simulink model "control"  (R2020a)
settings: Solver=FixedStepDiscrete  StartTime=0.0  StopTime=1  FixedStep=0.0005  RelTol=1e-3  EnableMultiTasking=on
undefined symbols (not defined in the file): acc_calmax1, acc_calmax2, acc_calmin1, acc_calmin2, akemancanshu, bre, bre_calmax, bre_calmin, ecucoder_acal, I_AN01_5K1, I_AN03_5V, I_AN04_5V, kd, ki, kp, leftmax, O_SW06_HS1A, rightmax, T_add, T_del, tiaoshi, zhiling
libraries: ec5744lib x252, canmsglib x92, simulink x5
(part 8 of 9)

== matlab function control/Subsystem/run/ctrl/Subsystem1/control_strategy/限滑/MPC/MPC/MPC左后/MPC_function ==
  data: x_k input; u_k output; U_init input
function u_k= Prediction(x_k,U_init)
% 定义状态矩阵 A, n*n 矩阵
A = 0;
% 定义输入矩阵 B, n*p 矩阵
R=0.2032;
FN=2058;
K=6.89;
B = R/(FN*K);
p = size(B,2);
% 定义Q矩阵，n*n 矩阵
Q = 100;
% 定义F矩阵，n*n 矩阵
F = 100;
% 定义R矩阵，p*p 矩阵
R = 1;
% 定义迭代次数和学习率
maxIterations = 5;
learningRate = 0.3;
N=5;%预测区间
n=size(A,1); % A是n*n矩阵,得到n
p=size(B,2); % B是n*p矩阵,得到p
M=[eye(n);zeros(N*n,n)]; % 初始化M矩阵,M矩阵是(N+1)n*n的
D=[0.17;zeros(N*n,n)];
C=zeros((N+1)*n,N*p); % 初始化C矩阵,这一步令它有(N+1)n*NP个0

% 定义M和C
tmp=eye(n); % 定义一个n*n 的 I 矩阵
    for i=1:N % 循环,i从1到N
        rows =i*n+(1:n); %定义当前行数,从i*n开始，共n行
        C(rows,:)=[tmp*B,C(rows-n, 1:end-p)]; %将c矩阵填满
        tmp= A*tmp; %每一次将tmp左乘一次A
        M(rows,:)=tmp; %将M矩阵写满
         D(rows,:)=0.17;
    end
    % 定义Q_bar和R_bar
    Q_bar = kron(eye(N),Q);
    Q_bar = blkdiag(Q_bar,F);
    R_bar = kron(eye(N),R);
    % 计算G,E,H
    G=M'*Q_bar*M; % G: n*n
    E=C'*Q_bar*M; % E: NP*n
    H=C'*Q_bar*C+R_bar; % NP*NP
 J=(D'*Q_bar*C)';
 L=E*x_k+J;
 U = U_init*ones(N*p,1); % NP x 1
%  options = optimoptions('quadprog', 'Algorithm', 'active-set');
%  U_k = quadprog(H,L, [], [], [], [], 0*ones(5,1), 1100*ones(5,1), 100*ones(5,1), options);
    % 梯度下降法求解最优二次规划问题
    G=size(U,1);
    S=zeros(G*maxIterations,1);
    for i = 1:maxIterations
        % 计算目标函数的梯度
        gradient = 2*H*U + 2*L;
        % 更新变量 U，并保持在 [0, 1100] 范围内
        U = U - learningRate * gradient;
        U = max(U, 0);
        U = min(U, 1100);
        O=(i-1)*maxIterations+(1:maxIterations);
        S(O,1)=U;
    end

 u_k = S(1:p,1); % 取第一个结果
end

== matlab function control/Subsystem/run/ctrl/Subsystem1/control_strategy/限滑/PID限滑/pid限滑与ABS ==
  data: slip input; throttle output; slip_ratio_limit input; brake output; u input
function [throttle, brake] = carPIDWithSlipControl(slip, slip_ratio_limit,u)
    % 赛车PID控制器参数
    kp = 0.2;
    ki = 0.1;
    kd = 0.01;
    
    % 状态变量
    persistent integral previous_error i
    
    % 初始化状态变量
    if isempty(integral)
        integral = 0;
        previous_error = 0;
        i=0;
    end
    
    % PID控制器计算
    error = 0.2 - slip;
    integral = integral + error*0.02;
    derivative = (error - previous_error)/0.02;
    
   k = kp * error + ki * integral + kd * derivative;
    if i<100
    
        output = u+k*u;
        if output>2000
            output=2000;
        end
    else
        output=u;
    end
    % 根据滑移率限制输出
  
    if slip > slip_ratio_limit
        brake = 0;%output;
        throttle = 0;
    else
        brake = 0;
        throttle = output;
    end
    
    % 保存上一个误差用于下次计算
    previous_error = error;

    i=i+1;
end

== matlab function control/Subsystem/run/ctrl/Subsystem1/control_strategy/限滑/PID限滑/pid限滑与ABS1 ==
  data: slip input; throttle output; slip_ratio_limit input; brake output; u input
function [throttle, brake] = carPIDWithSlipControl(slip, slip_ratio_limit,u)
    % 赛车PID控制器参数
    kp = 0.2;
    ki = 0.1;
    kd = 0.01;
    
    % 状态变量
    persistent integral previous_error i
    
    % 初始化状态变量
    if isempty(integral)
        integral = 0;
        previous_error = 0;
        i=0;
    end
    
    % PID控制器计算
    error = 0.2 - slip;
    integral = integral + error*0.02;
    derivative = (error - previous_error)/0.02;
    
   k = kp * error + ki * integral + kd * derivative;
    if i<100
    
        output = u+k*u;
        if output>2000
            output=2000;
        end
    else
        output=u;
    end
    % 根据滑移率限制输出
  
    if slip > slip_ratio_limit
        brake = 0;%output;
        throttle = 0;
    else
        brake = 0;
        throttle = output;
    end
    
    % 保存上一个误差用于下次计算
    previous_error = error;
    i=i+1;
end

== matlab function control/Subsystem/run/ctrl/Subsystem1/control_strategy/限滑/PID限滑/pid限滑与ABS2 ==
  data: slip input; throttle output; slip_ratio_limit input; brake output; u input
function [throttle, brake] = carPIDWithSlipControl(slip, slip_ratio_limit,u)
    % 赛车PID控制器参数
    kp = 0.2;
    ki = 0.1;
    kd = 0.01;
    
    % 状态变量
    persistent integral previous_error i
    
    % 初始化状态变量
    if isempty(integral)
        integral = 0;
        previous_error = 0;
        i=0;
    end
    
    % PID控制器计算
    error = 0.2 - slip;
    integral = integral + error*0.02;
    derivative = (error - previous_error)/0.02;
   k = kp * error + ki * integral + kd * derivative;
    if i<100
    
        output = u+k*u;
        if output>2000
            output=2000;
        end
    else
        output=u;
    end
    % 根据滑移率限制输出
  
    if slip > slip_ratio_limit
        brake = 0;%output;
        throttle = 0;
    else
        brake = 0;
        throttle = output;
    end
    
    % 保存上一个误差用于下次计算
    previous_error = error;
    i=i+1;
end

== matlab function control/Subsystem/run/ctrl/Subsystem1/control_strategy/限滑/PID限滑/pid限滑与ABS3 ==
  data: slip input; throttle output; slip_ratio_limit input; brake output; u input
function [throttle, brake] = carPIDWithSlipControl(slip, slip_ratio_limit,u)
    % 赛车PID控制器参数
    kp = 0.2;
    ki = 0.1;
    kd = 0.01;
    
    % 状态变量
    persistent integral previous_error i
    
    % 初始化状态变量
    if isempty(integral)
        integral = 0;
        previous_error = 0;
        i=0;
    end
    
    % PID控制器计算
    error = 0.2 - slip;
    integral = integral + error*0.02;
    derivative = (error - previous_error)/0.02;
    
   k = kp * error + ki * integral + kd * derivative;
    if i<100
    
        output = u+k*u;
        if output>2000
            output=2000;
        end
    else
        output=u;
    end
    % 根据滑移率限制输出
  
    if slip > slip_ratio_limit
        brake =0;% output;
        throttle = 0;
    else
        brake = 0;
        throttle = output;
    end
    
    % 保存上一个误差用于下次计算
    previous_error = error;
    i=i+1;
end

== matlab function control/Subsystem/Tx/TX控制器/速度/189左后/MATLAB Function5 ==
  data: v input; y output; angle input; vz input; model input
function y = fcn(v, angle, vz,model)
if(angle>3||angle<-3)&&model==3%4650000,4870000,4741002
    y=vz*594.06;
else
    y = v;
end

== matlab function control/Subsystem/run/ctrl/Subsystem1/control_strategy/限滑/PID限滑/计算油压 ==
  data: y1 input; p1 output; y2 input; y3 input; y4 input; p2 output; p3 output; p4 output
function [p1,p2,p3,p4]= fcn(y1,y2,y3,y4)
S=0.000491;
%p1 p2 p3 p4分别是左前、右前、左后、右后油压
p1=y1/(0.8*S)/1000;
p2=y2/(0.8*S)/1000;
p3=y3/(0.4*S)/1000;
p4=y4/(0.4*S)/1000;
% if p1<0
%     p1=0;
%     end
% if p2<0
%     p2=0;
%     end
% if p3<0
%     p3=0;
%     end
% if p4<0
%     p4=0;
% end

== matlab function control/Subsystem/run/ctrl/Subsystem1/control_strategy/限滑/Subsystem1/MATLAB Function2 ==
  data: u input; y output; mpc input; pid input; slip input; model input
function y = fcn(u,mpc,pid,slip,model)
if slip>0.8&&model~=6
    y=pid;
elseif slip>0.165&&slip<0.17
        y=mpc;
else
        y=u;
end
end

== matlab function control/Subsystem/run/ctrl/Subsystem1/control_strategy/限滑/Subsystem1/MATLAB Function3 ==
  data: u input; y output; mpc input; pid input; slip input; model input
function y = fcn(u,mpc,pid,slip,model)
if slip>0.8&&model~=6
    y=pid;
elseif slip>0.169&&slip<0.17
        y=mpc;
else
        y=u;
end
end

== matlab function control/Subsystem/run/ctrl/Subsystem1/control_strategy/限滑/Subsystem1/MATLAB Function4 ==
  data: u input; y output; mpc input; pid input; slip input; model input
function y = fcn(u,mpc,pid,slip,model)
if slip>0.8&&model~=6
    y=pid;
elseif slip>0.165&&slip<0.17
        y=mpc;
else
        y=u;
end
end

== matlab function control/Subsystem/run/ctrl/Subsystem1/control_strategy/限滑/Subsystem1/MATLAB Function5 ==
  data: u input; y output; mpc input; pid input; slip input; model input
function y = fcn(u,mpc,pid,slip,model)
if slip>0.8&&model~=6
    y=pid;
elseif slip>0.165&&slip<0.17
        y=mpc;
else
        y=u;
end
end

== matlab function control/Subsystem/Tx/TX控制器/速度1/184左前/MATLAB Function7 ==
  data: T input; y output; wurenyouya input; youya input; enable input; enable_1 input
function y = fcn(T, wurenyouya,youya, enable, enable_1)
 y = 0;
if wurenyouya>10||youya>500
    y = T;
else
    y=0;
end
if enable==0
    y=0;
end

== matlab function control/Subsystem/run/滑移率计算 ==
  data: vyouhou input; slipyuohou output; vyouqian input; vzouhou input; vzuoqian input; v input; slipyouqian output; slipzuohou output; slipzuoqian output; vmin input
function [slipyuohou,slipyouqian,slipzuohou,slipzuoqian] = fcn(vyouhou,vyouqian,vzouhou,vzuoqian,v,vmin)

    v1=vmin;
if v<0.1
    v1 = vmin;
else
    v1 = v;
end
slipyuohou= (vyouhou - v1) / vyouhou;
slipzuohou= (vzouhou - v1) / vzouhou;
slipyouqian= (vyouqian - v1) / vyouqian;
slipzuoqian= (vzuoqian - v1) / vzuoqian;
end

== matlab function control/Subsystem/Tx/TX控制器/速度1/188右后/MATLAB Function7 ==
  data: v input; youren input; T output; model input
function T = fcn(v,youren, model)
% if a>5
%     y = u;
% elseif a>3&&a<5
%     y=1200;
% else
%     y=800;
% end

if model==0||model==9||model==10   %有人模式，调试模式
    T=youren;
else                    %无人模式
   if v<6000*1.88e-3
     T=2100;
    elseif v>11000*1.88e-3
        T=800;
    else
        T=1100;
   end
end

== matlab function control/Subsystem/run/kalman_filter2 ==
  data: a_k_1 input; y output; v_k_1 input; v_k input; V_MIN input; model input
function y = fcn(a_k_1,v_k_1,v_k,V_MIN, model)
A=1;
H=1;
% x_real=v_k_1+0.02*a_k_1;%首先给出一个相应的估计值
% z=0;
% w=0;
% v=0;
% %%噪声信号
%     w=1*randn;
%     v=1*randn;
% %%状态方程
%     x_real=A*v_k_1+0.02*a_k_1+w;
% %%观测方程
%     z=H*x_real+v;
% persistent xhat;
%      % 初始化状态变量
%     if isempty(xhat)
%         xhat = V_MIN;
%     end

    z=H*v_k;
%%kalman_filter  根据上述得观测值来不断更新  
xhat=v_k;
xhat=v_k_1+0.02*a_k_1;%先验估计
Q=1;
R=0.01;
Pk=1;
Pk_bar=0;%先验协方差

    xhat_=v_k_1+0.02*a_k_1;%先验估计
    Pk_bar=A*Pk*A'+Q;
    Kk=Pk_bar*H'/(H*Pk_bar*H'+R);
    xhat= xhat_+ Kk*(z-H* xhat_);%最优估计值
    Pk=(1-Kk*H)*Pk_bar;
if v_k<0.1||model==0||model==9
    y=V_MIN;%即转轮时不使用惯导信息
elseif abs(xhat-v_k)>0.5
    y=v_k;
else
    y = xhat;
end
end

== matlab function control/Subsystem/Tx/TX控制器/速度/189左后/MATLAB Function6 ==
  data: v input; T output; a input
function T = fcn(v,a)
% if a>5
%     y = u;
% elseif a>3&&a<5
%     y=1200;
% else
%     y=800;
% end

if v<6000*1.88e-3
    T=2100;
elseif v>11000*1.88e-3
    T=800;
else
    T=1100;
end

== matlab function control/Subsystem/Tx/TX控制器/速度1/188右后/MATLAB Function6 ==
  data: T input; y output; wurenyouya input; youya input; enable input; enable_1 input
function y = fcn(T, wurenyouya,youya, enable, enable_1)
 y = 0;
if wurenyouya>10||youya>500
    y = T;
else
    y=0;
end
if enable==0
    y=0;
end

== matlab function control/Subsystem/Tx/TX控制器/速度1/189左后/MATLAB Function7 ==
  data: T input; y output; wurenyouya input; youya input; enable input; enable_1 input
function y = fcn(T, wurenyouya,youya, enable, enable_1)
 y = 0;
if wurenyouya>10||youya>500
    y = T;
else
    y=0;
end
if enable==0
    y=0;
end

== matlab function control/Subsystem/Tx/TX控制器/速度1/185右前/MATLAB Function7 ==
  data: T input; y output; wurenyouya input; youya input; enable input; enable_1 input
function y = fcn(T, wurenyouya,youya, enable, enable_1)
 y = 0;
if wurenyouya>10||youya>500
    y = T;
else
    y=0;
end
if enable==0
    y=0;
end

== matlab function control/Subsystem/Tx/TX控制器/速度1/184左前/能量回收功率限制/MATLAB Function ==
  data: youya input; T output; model input; status input; wurenyouya input
function T = fcn(youya, model, status, wurenyouya)
    if model == 0||model==10  %有人模式
        if youya>500
            T = -(youya-500)/4;%最大反扭1000
            if youya>4500
                T = -1000;
            end
        else
            T = 0;
        end
        
    elseif model~=0&&model~=9&&model~=2  %无人模式
        if wurenyouya>10
            T = -wurenyouya
            if status==5
                T=-1000;
            end  
           % T = -(wurenyouya-500)/4;%最大反扭1000
            %if wurenyouya>500&&status==5
             %   T = -1000;
            %end
        else
            T = 0;
        end
    else
        T = 0;
end

== matlab function control/Subsystem/Tx/TX控制器/速度1/184左前/能量回收功率限制/MATLAB Function1 ==
  data: er_T input; T output; Iq input; L_Iq input; L_er_T input
function T = fcn(er_T, Iq, L_Iq,L_er_T)
    if abs(Iq)>abs(L_Iq)
        T = -abs(L_er_T);

    else
        T = -abs(er_T);
    end

== matlab function control/Subsystem/Tx/TX控制器/速度1/188右后/能量回收功率限制/MATLAB Function ==
  data: youya input; T output; model input; status input; wurenyouya input
function T = fcn(youya, model, status, wurenyouya)
    if model == 0||model==10  %有人模式
        if youya>500
            T = -(youya-500)/4;%最大反扭1000
            if youya>4500
                T = -1000;
            end
        else
            T = 0;
        end
        
    elseif model~=0&&model~=9&&model~=2  %无人模式
        if wurenyouya>10
            T = -wurenyouya
        if status==5
                T=-1000;
            end  
           % T = -(wurenyouya-500)/4;%最大反扭1000
            %if wurenyouya>500&&status==5
             %   T = -1000;
            %end
        else
            T = 0;
        end
    else
        T = 0;
end

== matlab function control/Subsystem/Tx/TX控制器/速度1/188右后/能量回收功率限制/MATLAB Function1 ==
  data: er_T input; T output; Iq input; L_Iq input; L_er_T input
function T = fcn(er_T, Iq, L_Iq,L_er_T)
    if abs(Iq)>abs(L_Iq)
        T = -abs(L_er_T);

    else
        T = -abs(er_T);
    end

== matlab function control/Subsystem/Tx/TX控制器/速度/185右前/MATLAB Function2 ==
  data: enable input; enable_1 input; T input; TargetVelocity output; AMK_TorqueLimitPositive output; enable output; errorreset output; blnverteron output; CAN_dbcon output; v input
function [TargetVelocity,AMK_TorqueLimitPositive,enable,errorreset,blnverteron,CAN_dbcon]= fcn(enable,enable_1,T,v)
if (enable_1==0)
    TargetVelocity=0;
    enable=0;
    errorreset=1;
    blnverteron=0;
    CAN_dbcon=0;
    AMK_TorqueLimitPositive=0;
elseif (enable==0 && enable_1==1)
    TargetVelocity=2000;
    enable=1;
    errorreset=0;
    blnverteron=1;
    CAN_dbcon=1;
    AMK_TorqueLimitPositive=0;
elseif (enable==1 && enable_1==1)
    TargetVelocity=2000;
    enable=1;
    errorreset=0;
    blnverteron=1;
    CAN_dbcon=1;
    AMK_TorqueLimitPositive=T;
else
    TargetVelocity=0;
    enable=0;
    errorreset=1;
    blnverteron=0;
    CAN_dbcon=0;
    AMK_TorqueLimitPositive=0;
end

end

== matlab function control/Subsystem/Tx/TX控制器/速度1/189左后/能量回收功率限制/MATLAB Function ==
  data: youya input; T output; model input; status input; wurenyouya input
function T = fcn(youya, model, status, wurenyouya)
    if model == 0||model==10  %有人模式
        if youya>500
            T = -(youya-500)/4;%最大反扭1000
            if youya>4500
                T = -1000;
            end
        else
            T = 0;
        end
        
    elseif model~=0&&model~=9&&model~=2  %无人模式
        if wurenyouya>10
            T = -wurenyouya
            if status==5
                T=-1000;
            end
            
           % T = -(wurenyouya-500)/4;%最大反扭1000
            %if wurenyouya>500&&status==5
             %   T = -1000;
            %end
        else
            T = 0;
        end
    else
        T = 0;
end

== matlab function control/Subsystem/Tx/TX控制器/速度1/189左后/能量回收功率限制/MATLAB Function1 ==
  data: er_T input; T output; Iq input; L_Iq input; L_er_T input
function T = fcn(er_T, Iq, L_Iq,L_er_T)
    if abs(Iq)>abs(L_Iq)
        T = -abs(L_er_T);

    else
        T = -abs(er_T);
    end

== matlab function control/Subsystem/Tx/TX控制器/速度1/185右前/能量回收功率限制/MATLAB Function ==
  data: youya input; T output; model input; status input; wurenyouya input
function T = fcn(youya, model, status, wurenyouya)
    if model == 0||model==10  %有人模式
        if youya>500
            T = -(youya-500)/4;%最大反扭1000
            if youya>4500
                T = -1000;
            end
        else
            T = 0;
        end
        
    elseif model~=0&&model~=9&&model~=2  %无人模式
        if wurenyouya>10
            T = -wurenyouya
        if status==5
                T=-1000;
            end  
           % T = -(wurenyouya-500)/4;%最大反扭1000
            %if wurenyouya>500&&status==5
             %   T = -1000;
            %end
        else
            T = 0;
        end
    else
        T = 0;
end

== matlab function control/Subsystem/Tx/TX控制器/速度1/185右前/能量回收功率限制/MATLAB Function1 ==
  data: er_T input; T output; Iq input; L_Iq input; L_er_T input
function T = fcn(er_T, Iq, L_Iq,L_er_T)
    if abs(Iq)>abs(L_Iq)
        T = -abs(L_er_T);

    else
        T = -abs(er_T);
    end

== matlab function control/Subsystem/run/analog_input/无人意图转译/无人/Subsystem1/Subsystem/MATLAB Function ==
  data: u input; y output; v input; vd input
function y = fcn(u,v,vd)
persistent vv
if isempty(vv)
    vv=0;
end
if v-vd>0.1*v
    y=vv
else
    y=u;
end
vv=u;

== matlab function control/Subsystem/run/analog_input/MATLAB Function6 ==
  data: model input; y output
function y = fcn(model)
if model~=0||model~=10
    y = 1;
else
    y=0;
end

== matlab function control/Subsystem/Tx/TX控制器/速度/185右前/MATLAB Function4 ==
  data: u input; y output; zhidongesc input; zhidongebs input; huanting input
function y = fcn(u,zhidongesc,zhidongebs,huanting)
 y = u*594.06;
if zhidongesc>1800&&zhidongebs==2
    y = u*594.06;
end
if zhidongesc<1500&&zhidongebs==2
    y=0;
end
if huanting~=0
    y=0;
end

== matlab function control/Subsystem/Tx/TX控制器/速度/185右前/MATLAB Function5 ==
  data: v input; y output; angle input; vz input; model input
function y = fcn(v, angle, vz,model)
if(angle>3||angle<-3)&&model==3%4650000,4870000,4741002
    y=vz*594.06;
else
    y = v;
end

== matlab function control/Subsystem/Tx/TX控制器/速度/185右前/MATLAB Function6 ==
  data: v input; T output; a input
function T = fcn(v,a)
% if a>5
%     y = u;
% elseif a>3&&a<5
%     y=1200;
% else
%     y=800;
% end

if v<6000*1.88e-3
    T=2100;
elseif v>11000*1.88e-3
    T=800;
else
    T=1100;
end

== matlab function control/Subsystem/Tx/TX控制器/速度1/184左前/MATLAB Function ==
  data: u input; y output; zhidongesc input; zhidongebs input; huanting input
function y = fcn(u,zhidongesc,zhidongebs,huanting)
 y = u*594.06;
if zhidongesc>1800&&zhidongebs==2
    y = u*594.06;
end
if zhidongesc<1500&&zhidongebs==2
    y=0;
end
if huanting==0
    y=0;
end

== matlab function control/Subsystem/Tx/TX控制器/速度1/184左前/MATLAB Function1 ==
  data: v input; T output; a input
function T = fcn(v,a)
% if a>5
%     y = u;
% elseif a>3&&a<5
%     y=1200;
% else
%     y=800;
% end

if v<6000*1.88e-3
    T=2100;
elseif v>11000*1.88e-3
    T=800;
else
    T=1100;
end

== matlab function control/Subsystem/Tx/TX控制器/速度1/184左前/复位 ==
  data: enable input; enable_1 input; T input; TargetVelocity output; AMK_TorqueLimitPositive output; enable output; errorreset output; blnverteron output; CAN_dbcon output; v input
function [TargetVelocity,AMK_TorqueLimitPositive,enable,errorreset,blnverteron,CAN_dbcon]= fcn(enable,enable_1,T,v)
if (enable_1==0)
    TargetVelocity=0;
    enable=0;
    errorreset=1;
    blnverteron=0;
    CAN_dbcon=0;
    AMK_TorqueLimitPositive=0;
elseif (enable==0 && enable_1==1)
    TargetVelocity=0;
    enable=1;
    errorreset=0;
    blnverteron=1;
    CAN_dbcon=1;
    AMK_TorqueLimitPositive=0;
elseif (enable==1 && enable_1==1)
    TargetVelocity=v;
    enable=1;
    errorreset=0;
    blnverteron=1;
    CAN_dbcon=1;
    AMK_TorqueLimitPositive=T;
else
    TargetVelocity=0;
    enable=0;
    errorreset=1;
    blnverteron=0;
    CAN_dbcon=0;
    AMK_TorqueLimitPositive=0;
end

end

== matlab function control/Subsystem/Tx/TX控制器/速度/184左前/MATLAB Function2 ==
  data: enable input; enable_1 input; T input; TargetVelocity output; AMK_TorqueLimitPositive output; enable output; errorreset output; blnverteron output; CAN_dbcon output; v input
function [TargetVelocity,AMK_TorqueLimitPositive,enable,errorreset,blnverteron,CAN_dbcon]= fcn(enable,enable_1,T,v)
if (enable_1==0)
    TargetVelocity=0;
    enable=0;
    errorreset=1;
    blnverteron=0;
    CAN_dbcon=0;
    AMK_TorqueLimitPositive=0;
elseif (enable==0 && enable_1==1)
    TargetVelocity=2000;
    enable=1;
    errorreset=0;
    blnverteron=1;
    CAN_dbcon=1;
    AMK_TorqueLimitPositive=0;
elseif (enable==1 && enable_1==1)
    TargetVelocity=2000;
    enable=1;
    errorreset=0;
    blnverteron=1;
    CAN_dbcon=1;
    AMK_TorqueLimitPositive=T;
else
    TargetVelocity=0;
    enable=0;
    errorreset=1;
    blnverteron=0;
    CAN_dbcon=0;
    AMK_TorqueLimitPositive=0;
end

end

== matlab function control/Subsystem/Tx/TX控制器/速度1/184左前/MATLAB Function3 ==
  data: v input; y output; angle input; vz input; model input
function y = fcn(v, angle, vz,model)
if(angle>3||angle<-3)&&model==3%4650000,4870000,4741002
    y=vz*594.06;
else
    y = v;
end

== matlab function control/Subsystem/Tx/TX控制器/速度1/184左前/无人模式速度判断 ==
  data: u input; y output; zhidongesc input; zhidongebs input; huanting input
function y = fcn(u,zhidongesc,zhidongebs,huanting)
 y = u*594.06;
if zhidongesc>1800&&zhidongebs==2
    y = u*594.06;
end
if zhidongesc<1500&&zhidongebs==2
    y=0;
end
if huanting~=0
    y=0;
end

== matlab function control/Subsystem/Tx/TX控制器/速度1/184左前/有人无人速度转换 ==
  data: v input; y output; angle input; vz input; model input; zhidong input; T input; vk input
function y = fcn(v, angle, vz,model, zhidong, T, vk)
if model==0||model==9||model==10  %有人模式/无人检查（电气）
    if zhidong==0
       y=20000;
    else 
        y=0;
    end
else                    %无人模式
    if (angle>3||angle<-3)&&model==3 %4650000,4870000,4741002 大角度且八字
        y=vz*594.06;
    elseif T >10
        y=0;
        if vk<1
            y=vz*594.06;
        end
    else
        y = v;  
    end    
end

== matlab function control/Subsystem/Tx/TX控制器/速度1/184左前/有人无人扭矩转换 ==
  data: v input; youren input; T output; model input
function T = fcn(v,youren, model)
% if a>5
%     y = u;
% elseif a>3&&a<5
%     y=1200;
% else
%     y=800;
% end

if model==0||model==9||model==10   %有人模式，调试模式
    T=youren;
else                    %无人模式
   if v<6000*1.88e-3
     T=2100;
    elseif v>11000*1.88e-3
        T=800;
    else
        T=1100;
   end
end

== matlab function control/Subsystem/Tx/TX控制器/速度1/185右前/MATLAB Function ==
  data: u input; y output; zhidongesc input; zhidongebs input
function y = fcn(u,zhidongesc,zhidongebs)
 y = u*594.06;
if zhidongesc>1800&&zhidongebs==2
    y = u*594.06;
end
if zhidongesc<1500&&zhidongebs==2
    y=0;
end

== matlab function control/Subsystem/Tx/TX控制器/速度1/185右前/MATLAB Function1 ==
  data: v input; T output; a input
function T = fcn(v,a)
% if a>5
%     y = u;
% elseif a>3&&a<5
%     y=1200;
% else
%     y=800;
% end

if v<6000*1.88e-3
    T=2100;
elseif v>11000*1.88e-3
    T=800;
else
    T=1100;
end

== matlab function control/Subsystem/Tx/TX控制器/速度1/185右前/MATLAB Function2 ==
  data: enable input; enable_1 input; T input; TargetVelocity output; AMK_TorqueLimitPositive output; enable output; errorreset output; blnverteron output; CAN_dbcon output; v input
function [TargetVelocity,AMK_TorqueLimitPositive,enable,errorreset,blnverteron,CAN_dbcon]= fcn(enable,enable_1,T,v)
if (enable_1==0)
    TargetVelocity=0;
    enable=0;
    errorreset=1;
    blnverteron=0;
    CAN_dbcon=0;
    AMK_TorqueLimitPositive=0;
elseif (enable==0 && enable_1==1)
    TargetVelocity=0;
    enable=1;
    errorreset=0;
    blnverteron=1;
    CAN_dbcon=1;
    AMK_TorqueLimitPositive=0;
elseif (enable==1 && enable_1==1)
    TargetVelocity=v;
    enable=1;
    errorreset=0;
    blnverteron=1;
    CAN_dbcon=1;
    AMK_TorqueLimitPositive=T;
else
    TargetVelocity=0;
    enable=0;
    errorreset=1;
    blnverteron=0;
    CAN_dbcon=0;
    AMK_TorqueLimitPositive=0;
end

end

== matlab function control/Subsystem/Rx/lcu——receive/Subsystem1/Subsystem/MATLAB Function ==
  data: m input; y1 output; y2 output; y3 output
function [y1,y2,y3] = fcn(m)
V=zeros(1,3);
a=2;i=3;
while i>0
    V(1,i)=mod(m,a);
    m=fix(m/2);
    i=i-1;
end  
y1 = V(1,3);
y2=V(1,2);
y3=V(1,1);
end

== matlab function control/Subsystem/Rx/lcu——receive/Subsystem1/Subsystem/MATLAB Function1 ==
  data: u input; y output
function y = fcn(u)
if u==7
    y = 1;
else
    y=0;
end
end

== matlab function control/Subsystem/Tx/TX控制器/速度1/185右前/MATLAB Function3 ==
  data: v input; y output; angle input; vz input; model input
function y = fcn(v, angle, vz,model)
if (angle>3||angle<-3)&&model==3%4650000,4870000,4741002
    y=vz*594.06;
else
    y = v;
end

== matlab function control/Subsystem/Tx/TX控制器/速度1/185右前/MATLAB Function4 ==
  data: u input; y output; zhidongesc input; zhidongebs input; huanting input
function y = fcn(u,zhidongesc,zhidongebs,huanting)
 y = u*594.06;
if zhidongesc>1800&&zhidongebs==2
    y = u*594.06;
end
if zhidongesc<1500&&zhidongebs==2
    y=0;
end
if huanting~=0
    y=0;
end

== matlab function control/Subsystem/Tx/TX控制器/速度1/185右前/MATLAB Function5 ==
  data: v input; y output; angle input; vz input; model input; zhidong input; T input; vk input
function y = fcn(v, angle, vz,model, zhidong, T, vk)
if model==0||model==9||model==10  %有人模式/无人检查（电气）
    if zhidong==0
       y=20000;
    else 
        y=0;
    end
else                    %无人模式
    if (angle>3||angle<-3)&&model==3 %4650000,4870000,4741002 大角度和八字状态
        y=vz*594.06;
    elseif T >10
        y=0;
        if vk<1
            y=vz*594.06;
        end
    else
        y = v;
    end   
end

== matlab function control/Subsystem/Tx/TX控制器/速度1/185右前/MATLAB Function6 ==
  data: v input; youren input; T output; model input
function T = fcn(v,youren, model)
% if a>5
%     y = u;
% elseif a>3&&a<5
%     y=1200;
% else
%     y=800;
% end

if model==0||model==9||model==10   %有人模式，调试模式
    T=youren;
else                    %无人模式
   if v<6000*1.88e-3
     T=2100;
    elseif v>11000*1.88e-3
        T=800;
    else
        T=1100;
   end
end

== matlab function control/Subsystem/Tx/TX控制器/速度1/188右后/MATLAB Function ==
  data: u input; y output; zhidongesc input; zhidongebs input
function y = fcn(u,zhidongesc,zhidongebs)
 y = u*594.06;
if zhidongesc>1800&&zhidongebs==2
    y = u*594.06;
end
if zhidongesc<1500&&zhidongebs==2
    y=0;
end

== matlab function control/Subsystem/Tx/TX控制器/速度1/188右后/MATLAB Function1 ==
  data: v input; T output; a input
function T = fcn(v,a)
% if a>5
%     y = u;
% elseif a>3&&a<5
%     y=1200;
% else
%     y=800;
% end

if v<6000*1.88e-3
    T=2100;
elseif v>11000*1.88e-3
    T=800;
else
    T=1100;
end

== matlab function control/Subsystem/Tx/TX控制器/速度/184左前/MATLAB Function4 ==
  data: u input; y output; zhidongesc input; zhidongebs input; huanting input
function y = fcn(u,zhidongesc,zhidongebs,huanting)
 y = u*594.06;
if zhidongesc>1800&&zhidongebs==2
    y = u*594.06;
end
if zhidongesc<1500&&zhidongebs==2
    y=0;
end
if huanting~=0
    y=0;
end

== matlab function control/Subsystem/Tx/TX控制器/速度1/188右后/MATLAB Function2 ==
  data: enable input; enable_1 input; T input; TargetVelocity output; AMK_TorqueLimitPositive output; enable output; errorreset output; blnverteron output; CAN_dbcon output; v input
function [TargetVelocity,AMK_TorqueLimitPositive,enable,errorreset,blnverteron,CAN_dbcon]= fcn(enable,enable_1,T,v)
if (enable_1==0)
    TargetVelocity=0;
    enable=0;
    errorreset=1;
    blnverteron=0;
    CAN_dbcon=0;
    AMK_TorqueLimitPositive=0;
elseif (enable==0 && enable_1==1)
    TargetVelocity=0;
    enable=1;
    errorreset=0;
    blnverteron=1;
    CAN_dbcon=1;
    AMK_TorqueLimitPositive=0;
elseif (enable==1 && enable_1==1)
    TargetVelocity=v;
    enable=1;
    errorreset=0;
    blnverteron=1;
    CAN_dbcon=1;
    AMK_TorqueLimitPositive=T;
else
    TargetVelocity=0;
    enable=0;
    errorreset=1;
    blnverteron=0;
    CAN_dbcon=0;
    AMK_TorqueLimitPositive=0;
end

end

== matlab function control/Subsystem/Tx/TX控制器/速度1/188右后/MATLAB Function3 ==
  data: v input; y output; angle input; vz input; model input
function y = fcn(v, angle,vz,model)
if (angle>3||angle<-3)&&model==3%4650000,4870000,4741002
    y=vz*594.06;
else
    y = v;
end

== matlab function control/Subsystem/Tx/TX控制器/速度1/188右后/MATLAB Function4 ==
  data: u input; y output; zhidongesc input; zhidongebs input; huanting input
function y = fcn(u,zhidongesc,zhidongebs,huanting)
 y = u*594.06;
if zhidongesc>1800&&zhidongebs==2
    y = u*594.06;
end
if zhidongesc<1500&&zhidongebs==2
    y=0;
end
if huanting~=0
    y=0;
end

== matlab function control/Subsystem/Tx/TX控制器/速度1/188右后/MATLAB Function5 ==
  data: v input; y output; angle input; vz input; model input; zhidong input; T input; vk input
function y = fcn(v, angle, vz,model, zhidong, T, vk)
if model==0||model==9||model==10  %有人模式/无人检查（电气）
    if zhidong==0
       y=20000;
    else 
        y=0;
    end
else                    %无人模式
    if (angle>3||angle<-3)&&model==3 %4650000,4870000,4741002 大角度和八字状态
        y=vz*594.06;
    elseif T >10
        y=0;
        if vk<1
            y=vz*594.06;
        end
    else
        y = v;
    end    
end

== matlab function control/Subsystem/Tx/TX控制器/速度1/189左后/MATLAB Function6 ==
  data: v input; youren input; T output; model input
function T = fcn(v,youren, model)
% if a>5
%     y = u;
% elseif a>3&&a<5
%     y=1200;
% else
%     y=800;
% end

if model==0||model==9||model==10   %有人模式，调试模式
    T=youren;
else                    %无人模式
   if v<6000*1.88e-3
     T=2100;
    elseif v>11000*1.88e-3
        T=800;
    else
        T=1100;
   end
end

== matlab function control/Subsystem/Tx/TX控制器/速度1/189左后/MATLAB Function ==
  data: u input; y output; zhidongesc input; zhidongebs input
function y = fcn(u,zhidongesc,zhidongebs)
 y = u*594.06;
if zhidongesc>1800&&zhidongebs==2
    y = u*594.06;
end
if zhidongesc<1500&&zhidongebs==2
    y=0;
end

== matlab function control/Subsystem/Tx/TX控制器/速度1/189左后/MATLAB Function1 ==
  data: v input; T output; a input
function T = fcn(v,a)
% if a>5
%     y = u;
% elseif a>3&&a<5
%     y=1200;
% else
%     y=800;
% end

if v<6000*1.88e-3
    T=2100;
elseif v>11000*1.88e-3
    T=800;
else
    T=1100;
end

== matlab function control/Subsystem/Tx/TX控制器/速度1/189左后/MATLAB Function2 ==
  data: enable input; enable_1 input; T input; TargetVelocity output; AMK_TorqueLimitPositive output; enable output; errorreset output; blnverteron output; CAN_dbcon output; v input
function [TargetVelocity,AMK_TorqueLimitPositive,enable,errorreset,blnverteron,CAN_dbcon]= fcn(enable,enable_1,T,v)
if (enable_1==0)
    TargetVelocity=0;
    enable=0;
    errorreset=1;
    blnverteron=0;
    CAN_dbcon=0;
    AMK_TorqueLimitPositive=0;
elseif (enable==0 && enable_1==1)
    TargetVelocity=0;
    enable=1;
    errorreset=0;
    blnverteron=1;
    CAN_dbcon=1;
    AMK_TorqueLimitPositive=0;
elseif (enable==1 && enable_1==1)
    TargetVelocity=v;
    enable=1;
    errorreset=0;
    blnverteron=1;
    CAN_dbcon=1;
    AMK_TorqueLimitPositive=T;
else
    TargetVelocity=0;
    enable=0;
    errorreset=1;
    blnverteron=0;
    CAN_dbcon=0;
    AMK_TorqueLimitPositive=0;
end

end

== matlab function control/Subsystem/Tx/TX控制器/速度/184左前/MATLAB Function1 ==
  data: v input; T output; a input
function T = fcn(v,a)
% if a>5
%     y = u;
% elseif a>3&&a<5
%     y=1200;
% else
%     y=800;
% end

if v<6000*1.88e-3
    T=2100;
elseif v>11000*1.88e-3
    T=800;
else
    T=1100;
end

== matlab function control/Subsystem/Tx/TX控制器/速度/188右后/MATLAB Function1 ==
  data: v input; T output; a input
function T = fcn(v,a)
% if a>5
%     y = u;
% elseif a>3&&a<5
%     y=1200;
% else
%     y=800;
% end

if v<6000*1.88e-3
    T=2100;
elseif v>11000*1.88e-3
    T=800;
else
    T=1100;
end

== matlab function control/Subsystem/Tx/TX控制器/速度/184左前/MATLAB Function5 ==
  data: v input; y output; angle input; vz input; model input
function y = fcn(v, angle, vz,model)
if(angle>3||angle<-3)&&model==3%4650000,4870000,4741002
    y=vz*594.06;
else
    y = v;
end

== matlab function control/Subsystem/Rx/转向——receive1/Subsystem3/Subsystem/MATLAB Function ==
  data: u input; y output
function y = fcn(u)
y =   0.0003056 *u-208.4  ;
if u==683198
    y=0;
end

== matlab function control/Subsystem/Tx/TX控制器/速度1/189左后/MATLAB Function3 ==
  data: v input; y output; angle input; vz input; model input
function y = fcn(v, angle, vz,model)
if (angle>3||angle<-3)&&model==3%4650000,4870000,4741002
    y=vz*594.06;
else
    y = v;
end

== matlab function control/Subsystem/Tx/TX控制器/速度1/189左后/MATLAB Function4 ==
  data: u input; y output; zhidongesc input; zhidongebs input; huanting input
function y = fcn(u,zhidongesc,zhidongebs,huanting)
 y = u*594.06;
if zhidongesc>1800&&zhidongebs==2
    y = u*594.06;
end
if zhidongesc<1500&&zhidongebs==2
    y=0;
end
if huanting~=0
    y=0;
end

== matlab function control/Subsystem/Tx/TX控制器/速度1/189左后/MATLAB Function5 ==
  data: v input; y output; angle input; vz input; model input; zhidong input; T input; vk input
function y = fcn(v, angle, vz,model, zhidong, T, vk)
if model==0||model==9||model==10  %有人模式/无人检查（电气）
    if zhidong==0
       y=20000;
    else 
        y=0;
    end
else                    %无人模式
    if (angle>3||angle<-3)&&model==3 %4650000,4870000,4741002 大角度和八字状态
        y=vz*594.06;
    elseif T >10
        y=0;
        if vk<1
            y=vz*594.06;
        end
    else
        y = v;   
    end     
end

== matlab function control/Subsystem/run/kalman_filter1 ==
  data: a_k_1 input; y output; v_k_1 input; v_k input; V_MIN input; model input
function y = fcn(a_k_1,v_k_1,v_k,V_MIN, model)

    Z=v_k;%观测值
    %dt=0.02 ;%采样时间sampletime
    persistent X P F Q H R;%使函数退出后的计算值保持不变
    if isempty(X)% 检查是否是第一次运行，进行初始化
        X=0;%初始状态
        P=1;%状态协方差矩阵
        F=1;%状态转移矩阵
        Q=0.001;%状态转移协方差矩阵 
        H=1;%观测矩阵
        R=0.01;%观测噪声方差 

    end

    X_=v_k_1+0.01*a_k_1; %状态预测方程
    P_=F*P*F'+Q;%不确定性在各时刻的传递
    K=P_*H'/(H*P_*H'+R);%卡尔曼系数
    X=X_+K*(Z-H*X_);%状态更新
    P=(1-K*H)*P_;%噪声协方差矩阵更新
    
y=X;

if v_k<0.1||model==0||model==9||model==10
    y=V_MIN;  %即转轮时不使用惯导信息
elseif abs(X-v_k)>0.5
    y=v_k;
else
    y = X;
end
end

== matlab function control/Subsystem/run/LQR ==
  data: x input; y output
function y = fcn(x)
% A=[1 1;1 1];
% size(A,1);
% B=[1;1];
% P=size(B,2);
% ts=0.02;%离散时间的步长
% sys_d=c2d(ss(A,B),ts);%连续转离散系统函数，用于仿真代码
% x0=[1,1];%系统初始化
% x=x0;
% u0=0;
% u=u0;
% Q=[1 0 ;0 1];%系统权重
% S=[1 0;0 1];%终值权重
% R=0.1;%输入权重
% %定义系统运行步数
% k_steps = 100;
% %定义x._history雩矩阵,用于储存系统状态结果
% xhistory = zeros(n ,k_steps) ;
% %俘系统状态初始值赋值到x_history矩阵第一个位置
% xhistory (:,l)= x;
% %定义u_history需矩阵,用于储存系统输入结果,
% u_history = zeros(p,k_steps) ;
% %俘系统输入初始值赋值到u_history矩阵第一个位置
% u_history (:,1) = u;
% P_k = s;
% %计算最优反馈增益
% 
% 
% % 计算最优反馈增益
% for k = l : N
% % 计算F[N-k]
% F= inv(R+B'*P_k*B)*B'*P_k*A;
% 
% N= k_steps;
% P_k = s;
% % 计算最优反馈增益
% 
% P_k = (A-B*F)'*P_k*(A-B*F)+(F)'*R*(F)+Q;
% if k ==l
% F_N=F;
% else
% F_N=[F;F_N];
% end
% %仿真开始,建立for循环
% for k=l:k_steps
% u =-FN((k-1)*p+l:k*p ,:)*x;
% x= A*x+B*u ;
% %保存系统状态到预先定义矩阵的相应位置
% x_history(: ,k+l)=x;
% %保存系统输入到预先定义矩阵的相应位置
% u_history ( :,k)=u ;
% end
% 
% y=u;

== matlab function control/Subsystem/run/MATLAB Function ==
  data: u input; y output; u1 input; model input
function y = fcn(u,u1,model)
if ((u>0.8&&(model==0||model==10))||(u1>0.8))
    y = 1;
else
    y=0;
end

== matlab function control/Subsystem/run/MATLAB Function1 ==
  data: V_lon input; V_longitudinal output; V_lat input; theta_deg input; V_lateral output; V_MIN input
function [V_longitudinal, V_lateral] = calculateVelocities(V_lon, V_lat, theta_deg,V_MIN)
    % 将角度转换为弧度
    theta_rad = deg2rad(theta_deg);

    % 计算纵向速度和横向速度
    V_longitudinal_ = V_lon * sin(theta_rad) + V_lat * cos(theta_rad);
    if V_longitudinal_<0.2
         V_longitudinal=V_MIN;
    else
         V_longitudinal= V_longitudinal_;
    end
    V_lateral = V_lon * cos(theta_rad) -V_lat * sin(theta_rad);
end

== matlab function control/Subsystem/run/MATLAB Function2 ==
  data: u input; y output
function y = fcn(u)
if u>500
    y=1;
elseif u>1800
    y=2;
else
    y=0;
end

== matlab function control/Subsystem/run/analog_input/MATLAB Function ==
  data: u input; y output
function y = fcn(u)
if u==9
    y=1;
else
    y=0;
end

== matlab function control/Subsystem/run/analog_input/MATLAB Function1 ==
  data: u input; y output; a input
function y = fcn(u,a)
if u==1
    y=15;%%无人规则缓慢转轮
else
    y=a;
end
end

== matlab function control/Subsystem/Tx/TX控制器/速度/184左前/MATLAB Function6 ==
  data: v input; T output; a input
function T = fcn(v,a)
% if a>5
%     y = u;
% elseif a>3&&a<5
%     y=1200;
% else
%     y=800;
% end

if v<6000*1.88e-3
    T=2100;
elseif v>11000*1.88e-3
    T=800;
else
    T=1100;
end

== matlab function control/Subsystem/run/analog_input/MATLAB Function2 ==
  data: u input; y output; canok input
function y = fcn(u,canok)
if u==0%&&canok==1
    y=1;
else
    y=0;
end

== matlab function control/Subsystem/run/analog_input/MATLAB Function3 ==
  data: model input; y output; canok input; workstation input; v input
function y = fcn(model,canok,workstation,v)
if model~=0&&model~=10%%||canok==0
    y=1;
else
    y=0;
end
% if canok==0
%     y=0;
% end
%  if workstation<=0.1
%      y=0;
%  end
%  if v<0.5||v>18
%      y=0;
%  end

== matlab function control/Subsystem/Tx/TX控制器/速度/189左后/MATLAB Function1 ==
  data: v input; T output; a input
function T = fcn(v,a)
% if a>5
%     y = u;
% elseif a>3&&a<5
%     y=1200;
% else
%     y=800;
% end

if v<6000*1.88e-3
    T=2100;
elseif v>11000*1.88e-3
    T=800;
else
    T=1100;
end

== matlab function control/Subsystem/Tx/esc，ABS/MATLAB Function ==
  data: u input; y output
function y = fcn(u)
if u~=0&&u~=9&&u~=2
    y=1;
else
    y=0;
end

== matlab function control/Subsystem/run/analog_input/MATLAB Function4 ==
  data: u input; y output; a input
function y = fcn(u,a)
if u==5
    y=0;
else
    y=a;
end
end

== matlab function control/Subsystem/Rx/工作站/Subsystem3/Subsystem/MATLAB Function ==
  data: u input; y output; CANOK_20 input
function y = fcn(u,CANOK_20)
if CANOK_20==0
    y=0;
else
    y=u;
end

== matlab function control/Subsystem/run/analog_input/MATLAB Function5 ==
  data: u input; y output; model input; y6 output
function [y,y6] = fcn(u,model)
if model==8
    y = 0;
    y6=u;
else
    y=u;
    y6=0;
end
if y~=0&&y6~=0
    y=0;
    y6=0;
end
    
end

== matlab function control/Subsystem/Rx/工作站/Subsystem3/Subsystem/MATLAB Function1 ==
  data: u input; y output; CANOK_20 input
function y = fcn(u,CANOK_20)
% if CANOK_20==0
%     y=0;
% else
    y=u;
% end

== matlab function control/Subsystem/Tx/转向/MATLAB Function1 ==
  data: model input; y output; status input
function y = fcn(model,status)
if (model==1||model==3||model==4||model==5||model==6||model==7||model==8)&&(status==3||status==4||status==5)
    y=1;
else
    y=0;
end
if model==8
    y=1;
else
    y=y;
end

== matlab function control/Subsystem/Rx/lcu——receive/MATLAB Function ==
  data: m input; enable_185 output; enable_185_1 output; enable_188 output; enable_188_1 output; enable_184 output; enable_184_1 output; enable_189 output; enable_189_1 output
%八位无符号数
function [enable_185,enable_185_1,enable_188,enable_188_1,enable_184,enable_184_1,enable_189,enable_189_1] = ErJinZhi(m)
V=zeros(1,8);
a=2;i=8;
while i>0
    V(1,i)=mod(m,a);
    m=fix(m/2);
    i=i-1;
end    
enable_185=V(1,1);%右前
enable_185_1=V(1,2);
enable_188=V(1,3);%右后
enable_188_1=V(1,4);
enable_184=V(1,5);
enable_184_1=V(1,6);%左前
enable_189=V(1,7);
enable_189_1=V(1,8);%左后
end

== matlab function control/Subsystem/Tx/转向/转向换算/MATLAB Function ==
  data: biaozhi1 output; baocuo input
function biaozhi1  = fcn(baocuo)
persistent i;
     % 初始化状态变量
    if isempty(i)
        i = 1;
    end
    if baocuo==1
        i=1;
    end
    if i>4
        biaozhi1=1;
    else
        biaozhi1=0;       
    end
i=i+1;
end

== matlab function control/Subsystem/Tx/转向/转向换算/Subsystem/MATLAB Function ==
  data: steer output; y output; x input; canok input; baocuo input; k input; d input; rm input; lm input
function [steer,y] = fcn(x,canok,baocuo,k,d,rm,lm)
  persistent i previoussteer;
     % 初始化状态变量
     rm=rm-3000;
     lm=lm+3000;
    if isempty(i)
        i = 0;
    end
    if isempty(previoussteer)
        previoussteer= d;
    end
    if i>0.2     
        steer= k *x+d ;
%         if x==0
%             steer=25092;
%         end
          if steer>rm
              steer=rm;
          end
          if steer<lm
              steer=lm;
          end
    else
        steer=d;
    end
    if canok==0
        steer=previoussteer;
    end
    if baocuo==1
        steer=previoussteer;
    end
    i=i+0.02;
  persistent time  a b;
     % 初始化状态变量
    if isempty(time)
        time = 0;
   
        a=5;
        b=10;
    end
    if baocuo==1
        time=-4;
    end
    if mod(abs(time), 2) == 0
        result = 1;
    else
        result = 0;
    end
    if time<b&&result==0
    y=6;
 
    elseif time<b&&result==1
    y=15;
  
    elseif time>=b
        if result==1
            y=79;
        else
            y=63;
        end
    else
        y=6;
    end   
    time=time+1;
    previoussteer=steer;
%     
%       persistent time1;
%      % 初始化状态变量
%     if isempty(time1)
%         time1 = 0;
%     end
%     if mod(time1, 2) == 0
%         result1 = 1;
%     else
%         result1 = 0;
%     end
%     if time1<2
%     y=6;
%  
%     elseif time1>=2&&time1<4
%     y=15;
%   
%     elseif time1>=4
%         if result1==1
%             y=79;
%         else
%             y=63;
%         end
%     else
%         y=6;
%     end   
%     time1=time1+1;
   
end

== matlab function control/Subsystem/Rx/工作站/Subsystem3/Subsystem/MATLAB Function2 ==
  data: u input; y output; CANOK_20 input
function y = fcn(u, CANOK_20)


% 初始化位数计数
num_digits = 0; 
% 处理0的情况
if u == 0
    num_digits = 1;
else
    % 计算位数
    num = abs(u);
    while num > 0
        num = floor(num / 10);
        num_digits = num_digits + 1;
    end
end
    divisor = 10 ^ num_digits;
    decimal = u / divisor;
    if u>0
        y=decimal;
    else
        y=-decimal;
    end
    if CANOK_20==0
    y=0;
    end
end

== matlab function control/Subsystem/Rx/工作站/Subsystem3/Subsystem/MATLAB Function3 ==
  data: u input; y output; CANOK_20 input
function y = fcn(u,CANOK_20)

% 初始化位数计数
num_digits = 0; 
% 处理0的情况
if u == 0
    num_digits = 1;
else
    % 计算位数
    num = abs(u);
    while num > 0
        num = floor(num / 10);
        num_digits = num_digits + 1;
    end
end
    divisor = 10 ^ num_digits;
    decimal = u / divisor;
    if u>0
        y=decimal;
    else
        y=-decimal;
    end
%     if CANOK_20==0
%     y=0;
%     end
end

== matlab function control/Subsystem/Rx/283 285左前/Subsystem2/Subsystem/MATLAB Function ==
  data: u input; y output
function y = fcn(u)

y = u/594.06;

== matlab function control/Subsystem/Rx/284 286右前/Subsystem2/Subsystem/MATLAB Function ==
  data: u input; y output
function y = fcn(u)


y = u/594.06;

== matlab function control/Subsystem/Rx/288 290左后/Subsystem2/Subsystem/MATLAB Function ==
  data: u input; y output
function y = fcn(u)


y = u/594.06;

== matlab function control/Subsystem/run/analog_input/无人意图转译/无人/Subsystem1/Desired/MATLAB Function ==
  data: u input; y output
function y = fcn(u)
  % 状态变量
    persistent i
    % 初始化状态变量
    if isempty(i)
       
        i=0;
    end
    y=(u-i)*50;
    if y>23.2
        y=23.2;
    end
    i=u;

== matlab function control/Subsystem/run/analog_input/无人意图转译/无人/Subsystem1/Desired/MATLAB Function1 ==
  data: u input; y output
function y = fcn(u)

 persistent i
    % 初始化状态变量
    if isempty(i)
       
        i=0;
    end
    y=(u-i)*50;
    i=u;

== matlab function control/Subsystem/Tx/TX控制器/扭矩/TEST/MATLAB Function ==
  data: u input; y output
function y = fcn(u)
if u~=0%%&&u~=6
    y=1;
else
    y=0;
end

== matlab function control/Subsystem/Tx/TX控制器/MATLAB Function ==
  data: v input; model input; v_k input; ysudu output; yniuju output
function [ysudu,yniuju] = fcn(v,model,v_k)
if v>25
    yniuju=1;
    ysudu=0;
else
    yniuju=0;
    ysudu=1;
end

%if v_k<0.5||v_k>18
%     yniuju=0;
%     ysudu=1;
%end
if model==9
    yniuju=1;
    ysudu=0;
end
if model==0
    yniuju=1;
    ysudu=0;
end
if yniuju==ysudu
    yniuju=0;
    ysudu=0;
end

== matlab function control/Subsystem/Rx/转向——receive编码器/Subsystem3/Subsystem/MATLAB Function ==
  data: u input; y output
function y = fcn(u)
if u<180
    y=-u/4.1;
else
    y=(360-u)/4.1;
end

== matlab function control/Subsystem/Tx/转向/转向换算/Subsystem/转向修正 ==
  data: steerbianmaqi input; steerangle input; steernew output; steer input; error output; k input; KP input; KI input; KD input; model input
function [ steernew,error]  = carPIDWithSlipControl(steerbianmaqi,steerangle,steer,k,KP,KI,KD,model)
    % 赛车PID控制器参数
    if k==0
%         kp=1.25;
%         ki=0.27;
%         kd=0.6;
%         kp = 1.5;
%         ki = 0.4;
%         kd = 0.65;
%    kp = 1.2;
%     ki = 0.25;
%     kd = 0.55;
        kp = 0.4;
        ki = 0.13;
        kd = 0.3;
     else
        kp=KP;
        ki=KI;
        kd=KD;
    end
    if (model==1)&&(steer<5)
        kp=0.8;
        ki=0.1;
        kd=0.15;
    end
%     else
%         kp=KP;
%         ki=KI;
%         kd=KD;
%     end
    %kp = 1.2;
    %ki = 0.25;
    %kd = 0.55;
    % 状态变量
    persistent integral previous_error  presteer preerrorbianmaqi
    
    % 初始化状态变量
    if isempty(integral)
        integral = 0;
        previous_error = 0;
       presteer=0;
        preerrorbianmaqi=0;
    end
    errorbianmaqi=steerangle-steerbianmaqi;
    % PID控制器计算
    error = steer - steerbianmaqi;
    integral = integral + error*0.02;
    derivative = (error - previous_error)/0.02;
    

%     if abs(steer)<0.5%零点消除抖震
%         kp=0;
%         ki=0;
%         kd=0;
%     end
        
   
    K= kp * error + ki * integral + kd * derivative;
   if K<0.05%消抖
       K=0;
   end
   
        steernew =steer+K;

    if (steer*presteer<0)
        integral=0;
        if (abs(error)>1.3)&&(abs(steer)<5)&&(abs(steer-steerbianmaqi)>3)&&(model==1)
            if steer>0
                steernew=7;
            end
            if steer<0
                steernew=-7;
            end
        end
    end
    % 保存上一个误差用于下次计算
    previous_error = error;
     preerrorbianmaqi= errorbianmaqi;
     presteer=steer;
end

== matlab function control/Subsystem/Tx/Toworkstation/转向/MATLAB Function ==
  data: u input; y output
function y = fcn(u)
if u==9
    y=1;
else
    y=0;
end

== matlab function control/Subsystem/Tx/Toworkstation/转向/Subsystem/MATLAB Function ==
  data: biaozhi1 output
function biaozhi1  = fcn
persistent i;
     % 初始化状态变量
    if isempty(i)
        i = 1;
    end
    if i>16
        biaozhi1=1;
    else
        biaozhi1=0;
    end
    i=i+1;
end

== matlab function control/Subsystem/run/analog_input/无人意图转译/无人/Subsystem1/MATLAB Function ==
  data: u input; y output; u2 input
function y = fcn(u,u2)

y = u-u2;

== matlab function control/Subsystem/run/analog_input/无人意图转译/无人/Subsystem1/Desired/MATLAB Function2 ==
  data: u1 input; y output; u2 input; u3 input; u4 input; u5 input; model input; v1 input; v2 input; v3 input; v4 input; v5 input; V output
function [y,V] = fcn(u1,u2,u3,u4,u5,model,v1,v2,v3,v4,v5)
y=u1;
V=v1;
if u1>5&&u1<=10
    y=(u1+u2+u3)/3;
    V=(v1+v2+v3)/3;
end
if u1>10
    y=(u1+u2+u3+u4+u5)/5;
    V=(v1+v2+v3+v4+v5)/5;
end
if model==1
    y=u1;
    V=v1;
end
if model==0
    y=0;
    V=0;
end
if u1<0
    y=u1;
    V=v1;
end

== matlab function control/Subsystem/Tx/TX控制器/速度/188右后/MATLAB Function2 ==
  data: enable input; enable_1 input; T input; TargetVelocity output; AMK_TorqueLimitPositive output; enable output; errorreset output; blnverteron output; CAN_dbcon output; v input
function [TargetVelocity,AMK_TorqueLimitPositive,enable,errorreset,blnverteron,CAN_dbcon]= fcn(enable,enable_1,T,v)
if (enable_1==0)
    TargetVelocity=0;
    enable=0;
    errorreset=1;
    blnverteron=0;
    CAN_dbcon=0;
    AMK_TorqueLimitPositive=0;
elseif (enable==0 && enable_1==1)
    TargetVelocity=2000;
    enable=1;
    errorreset=0;
    blnverteron=1;
    CAN_dbcon=1;
    AMK_TorqueLimitPositive=0;
elseif (enable==1 && enable_1==1)
    TargetVelocity=2000;
    enable=1;
    errorreset=0;
    blnverteron=1;
    CAN_dbcon=1;
    AMK_TorqueLimitPositive=T;
else
    TargetVelocity=0;
    enable=0;
    errorreset=1;
    blnverteron=0;
    CAN_dbcon=0;
    AMK_TorqueLimitPositive=0;
end

end

== matlab function control/Subsystem/run/analog_input/无人意图转译/无人/Subsystem1/MATLAB Function3 ==
  data: u input; y1 output; y2 output; v input; vd input; ade input; adede input; adedede input
function [y1,y2] = fcn(u,v,vd,ade,adede,adedede)
persistent i
    if isempty(i)
       
        i=0;
    end
dota=(u-i);
if v-vd>5
    u=0;
end
if u>=0
    if dota>1
    y1=(u+i+ade+adede+adedede)/5;
    else
    y1=u;
    end
    y2=0;
else
    y1=0;
    y2=u;
end

if u<0
    y2=u;
end
i=u;
end

== matlab function control/Subsystem/Rx/lcu——receive/Subsystem1/Subsystem/MATLAB Function2 ==
  data: u input; y output
function y = fcn(u)
% if(u==1||u==4)
if(u==4)
    y=1;
else
    y=0;
end

== matlab function control/Subsystem/Rx/工作站/Subsystem3/Subsystem/MATLAB Function4 ==
  data: u input; y output; nengbunengpao input; model input

function y = fcn(u,nengbunengpao,model)
if nengbunengpao==1
    y = u;
else
    y=0;
end
if model==6
    y=u;
else
    y=y;
end
